simulink model "calibJointTorqueSens"  (Simulink 8.3)
settings: Solver=ode45  StartTime=0.0  StopTime=10.0  RelTol=1e-3
undefined symbols (not defined in the file or in its folder): calibDelta, CONFIG, WBT_robotName
undefined symbols (not defined in the file): FRAMES
libraries: WBToolboxLibrary x12
settings Model: Creator=gabri  LastModifiedBy=gabri
settings DataIOCC: SignalLoggingSaveFormat=Dataset
settings DebuggingCC: UnderspecifiedInitializationDetection=Simplified  StateNameClashWarn=none
settings GRTTargetCC: CombineOutputUpdateFcns=on  GRTInterface=off

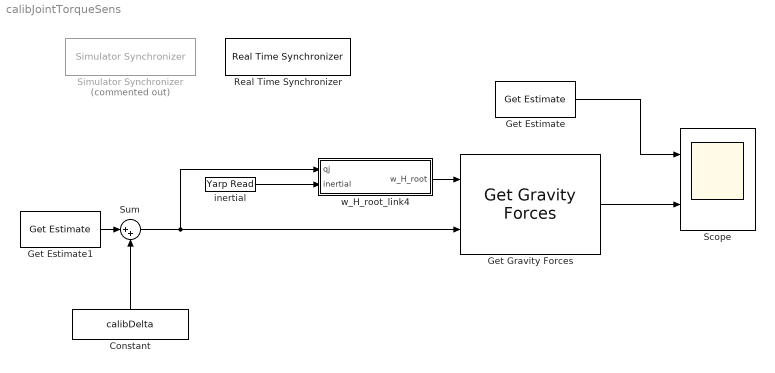
== system calibJointTorqueSens ==
  Constant : Constant  Value=calibDelta
  Get Estimate : WBToolboxLibrary/wholeBodyStates/Get Estimate  estimateType=Joints Torque  robotName=WBT_robotName  localName=WBT_modelName  wbiFile=WBT_wbiFilename  wbiList=WBT_wbiList
  Get Estimate1 : WBToolboxLibrary/wholeBodyStates/Get Estimate  estimateType=Joints Position  robotName=WBT_robotName  localName=WBT_modelName  wbiFile=WBT_wbiFilename  wbiList=WBT_wbiList
  Get Gravity Forces : WBToolboxLibrary/wholeBodyModel/Dynamics/Get Gravity Forces  robotName=WBT_robotName  localName=WBT_modelName  wbiFile=WBT_wbiFilename  wbiList=WBT_wbiList  explicitGravity=off
  Real Time Synchronizer : WBToolboxLibrary/Utilities/Real Time Synchronizer  period=0.01
  Scope : Scope  NumInputPorts=2
      settings: YMin=-5~-5  YMax=5~5
  Simulator Synchronizer : WBToolboxLibrary/Utilities/Simulator Synchronizer  Commented=on  period=0.01  serverPortName='/clock/rpc'  clientPortName='/WBT_synchronizer/rpc:o'
  Sum : Sum  Inputs=|++
  inertial : WBToolboxLibrary/Utilities/Yarp Read  portName=PORTS.IMU  signalSize=12  blocking=off  timestamp=off  autoconnect=on  errorOnConnection=off
  w_H_root_link4 : Subsystem  mask{link_name=FRAMES.BASE}
      mask prompts: link_name "link name"
      mask help:
      | This block evaluates the homogeneous transformation between the world and the root link, i.e. ^wH_b. It assumes that the link specified by the variable 'link_name' has a constant position
      | w.r.t. an inertial frame, but it can rotate arbitrarily. This rotation is retrived from the IMU sensor.
      mask Display:
      | str = strrep(link_name, '_','\_');
      | port_label('output',1,['{}^{',str '}H_{root}'],'texmode','on')
      | clear str;
      | 
      | port_label('input',1,'q_j','texmode','on')
      | 
      | port_label('input',2,'inertial','texmode','on')
  wires:
  w_H_root_link4/1(w_H_root) -> Get Gravity Forces/1
  inertial/1 -> w_H_root_link4/2(inertial)
  Get Estimate1/1 -> Sum/1
  Sum/1 -> w_H_root_link4/1(qj), Get Gravity Forces/2
  Constant/1 -> Sum/2
  Get Gravity Forces/1 -> Scope/2
  Get Estimate/1 -> Scope/1

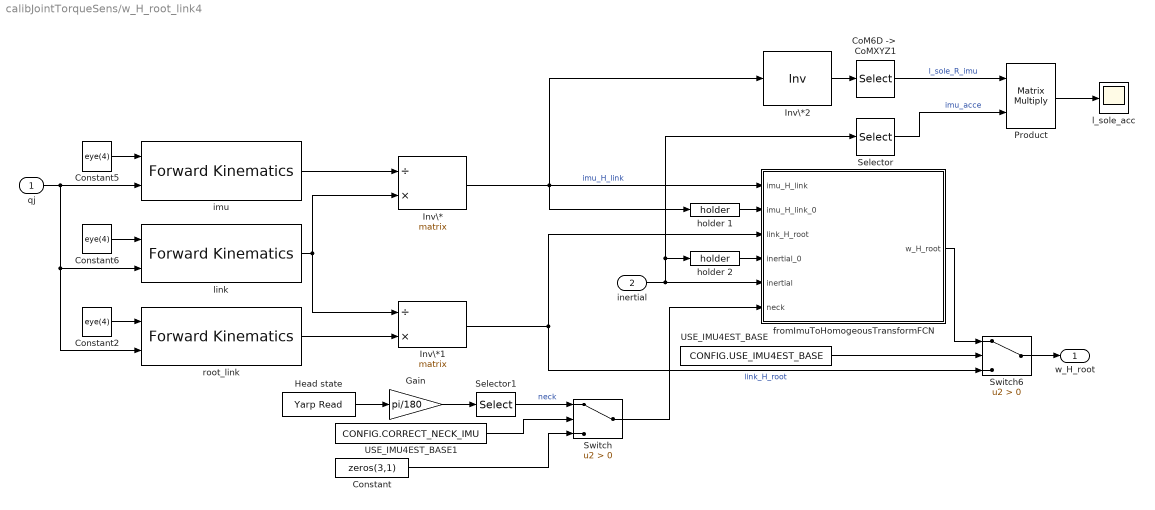
== system calibJointTorqueSens/w_H_root_link4 ==
  qj : Inport
  inertial : Inport  Port=2
  "CoM6D ->  CoMXYZ1" : Selector  NumberOfDimensions=2  InputPortWidth=7  IndexOptions=Index vector (dialog),Index vector (dialog)  Indices=[1 2 3],[1 2 3]  OutputSizes=1,1
  Constant : Constant  Value=zeros(3,1)
  Constant2 : Constant  Value=eye(4)
  Constant5 : Constant  Value=eye(4)
  Constant6 : Constant  Value=eye(4)
  Gain : Gain  Gain=pi/180
  Head state : WBToolboxLibrary/Utilities/Yarp Read  portName=[WBT_robotName, '/head/state:o']  signalSize=6  blocking=off  timestamp=off  autoconnect=on  errorOnConnection=off
  Inv\* : Product  Inputs=/*  Multiplication=Matrix(*)
  Inv\*1 : Product  Inputs=/*  Multiplication=Matrix(*)
  Inv\*2 : Product  Inputs=/  Multiplication=Matrix(*)
  Product : Product  Multiplication=Matrix(*)
  Selector : Selector  InputPortWidth=12  Indices=[4 5 6 ]
  Selector1 : Selector  InputPortWidth=6  Indices=[1:3]
  Switch : Switch  Criteria=u2 > Threshold
  Switch6 : Switch  Criteria=u2 > Threshold
  USE_IMU4EST_BASE : Constant  Value=CONFIG.USE_IMU4EST_BASE
  USE_IMU4EST_BASE1 : Constant  Value=CONFIG.CORRECT_NECK_IMU
  fromImuToHomogeousTransformFCN : MATLAB Function  TreatAsAtomicUnit=on
  holder 1 : WBToolboxLibrary/Utilities/holder 
  holder 2 : WBToolboxLibrary/Utilities/holder 
  imu : WBToolboxLibrary/wholeBodyModel/Kinematics/Forward Kinematics  frameName=FRAMES.IMU  robotName=WBT_robotName  localName=WBT_modelName  wbiFile=WBT_wbiFilename  wbiList=WBT_wbiList
  l_sole_acc : Scope
      settings: ShowLegends=on  TimeRange=60  YMin=-4.47309  YMax=14.2668
  link : WBToolboxLibrary/wholeBodyModel/Kinematics/Forward Kinematics  frameName=link_name  robotName=WBT_robotName  localName=WBT_modelName  wbiFile=WBT_wbiFilename  wbiList=WBT_wbiList
  root_link : WBToolboxLibrary/wholeBodyModel/Kinematics/Forward Kinematics  frameName=FRAMES.BASE  robotName=WBT_robotName  localName=WBT_modelName  wbiFile=WBT_wbiFilename  wbiList=WBT_wbiList
  w_H_root : Outport
  wires:
  Constant5/1 -> imu/1
  Inv\*/1 -> Inv\*2/1, holder 1/1, fromImuToHomogeousTransformFCN/1(imu_H_link)  "imu_H_link"
  imu/1 -> Inv\*/1
  Constant6/1 -> link/1
  Inv\*1/1 -> Switch6/3, fromImuToHomogeousTransformFCN/3(link_H_root)  "link_H_root"
  link/1 -> Inv\*/2, Inv\*1/1
  inertial/1 -> Selector/1, holder 2/1, fromImuToHomogeousTransformFCN/5(inertial)
  Switch6/1 -> w_H_root/1
  USE_IMU4EST_BASE/1 -> Switch6/2
  fromImuToHomogeousTransformFCN/1(w_H_root) -> Switch6/1
  Constant2/1 -> root_link/1
  qj/1 -> root_link/2, link/2, imu/2
  root_link/1 -> Inv\*1/2
  holder 1/1 -> fromImuToHomogeousTransformFCN/2(imu_H_link_0)
  holder 2/1 -> fromImuToHomogeousTransformFCN/4(inertial_0)
  Inv\*2/1 -> "CoM6D ->  CoMXYZ1"/1
  "CoM6D ->  CoMXYZ1"/1 -> Product/1  "l_sole_R_imu"
  Selector/1 -> Product/2  "imu_acce"
  Product/1 -> l_sole_acc/1
  Head state/1 -> Gain/1
  Selector1/1 -> Switch/1  "neck"
  USE_IMU4EST_BASE1/1 -> Switch/2
  Switch/1 -> fromImuToHomogeousTransformFCN/6(neck)
  Gain/1 -> Selector1/1
  Constant/1 -> Switch/3

== matlab function w_H_root_link4/fromImuToHomogeousTransformFCN ==
  data: imu_H_link input double; imu_H_link_0 input double; link_H_root input double; inertial_0 input double; inertial input double; neck input double; w_H_root output double; CONFIG parameter double
function w_H_root = fromBaseToWorldWithImuFCN(imu_H_link,imu_H_link_0,link_H_root,inertial_0,inertial,neck,CONFIG)
%#codegen
w_H_root = fromBaseToWorldWithImu(imu_H_link,imu_H_link_0,link_H_root,inertial_0,inertial,neck,CONFIG);
